simulink model "mass_spring_damper_control"  (R2022a)
settings: Solver=VariableStepAuto  StartTime=0.0  StopTime=10.0  MaxStep=1e-2  RelTol=1e-3
InitFcn:
  | start;
values from neighbouring files (symbols this model uses):
  d = 1    [start.m]
  dy0 = 0    [start.m]
  k = 2    [start.m]
  m = 1    [start.m]
  y0 = 0    [start.m]
settings Model: Creator=mathe  LastModifiedBy=mathe

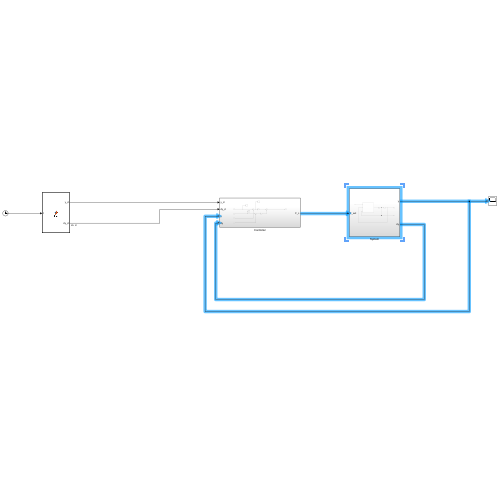
[thumbnail: Simulink's stored preview of the top-level diagram]
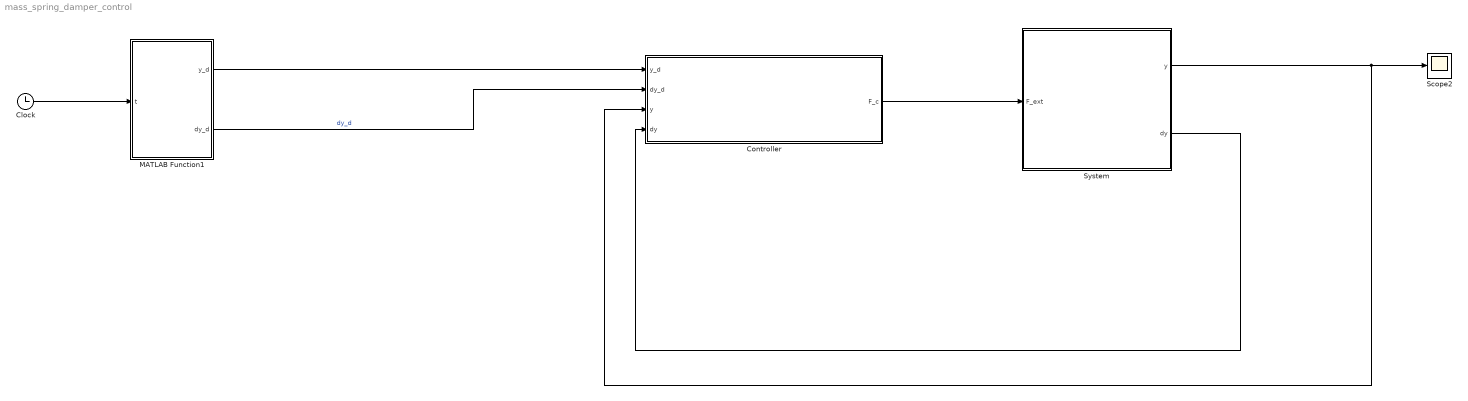
== system mass_spring_damper_control ==
  Clock : Clock
  Controller : Subsystem
  MATLAB Function1 : MATLAB Function  TreatAsAtomicUnit=on
  Scope2 : Scope
  System : Subsystem
  wires:
  Clock/1 -> MATLAB Function1/1(t)
  System/1(y) -> Controller/3(y), Scope2/1
  MATLAB Function1/1(y_d) -> Controller/1(y_d)
  System/2(dy) -> Controller/4(dy)
  MATLAB Function1/2(dy_d) -> Controller/2(dy_d)  "dy_d"
  Controller/1(F_c) -> System/1(F_ext)

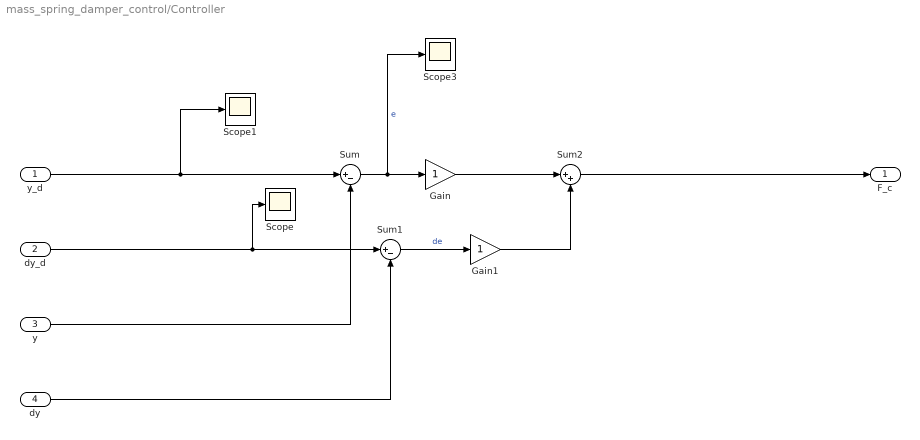
== system mass_spring_damper_control/Controller ==
  y_d : Inport
  dy_d : Inport  Port=2
  y : Inport  Port=3
  dy : Inport  Port=4
  Gain : Gain
  Gain1 : Gain
  Scope : Scope
  Scope1 : Scope
  Scope3 : Scope
  Sum : Sum  Inputs=|+-
  Sum1 : Sum  Inputs=|+-
  Sum2 : Sum  Inputs=|++
  F_c : Outport
  wires:
  Gain1/1 -> Sum2/2
  dy_d/1 -> Scope/1, Sum1/1
  Sum/1 -> Scope3/1, Gain/1  "e"
  Gain/1 -> Sum2/1
  y_d/1 -> Scope1/1, Sum/1
  Sum2/1 -> F_c/1
  Sum1/1 -> Gain1/1  "de"
  dy/1 -> Sum1/2
  y/1 -> Sum/2

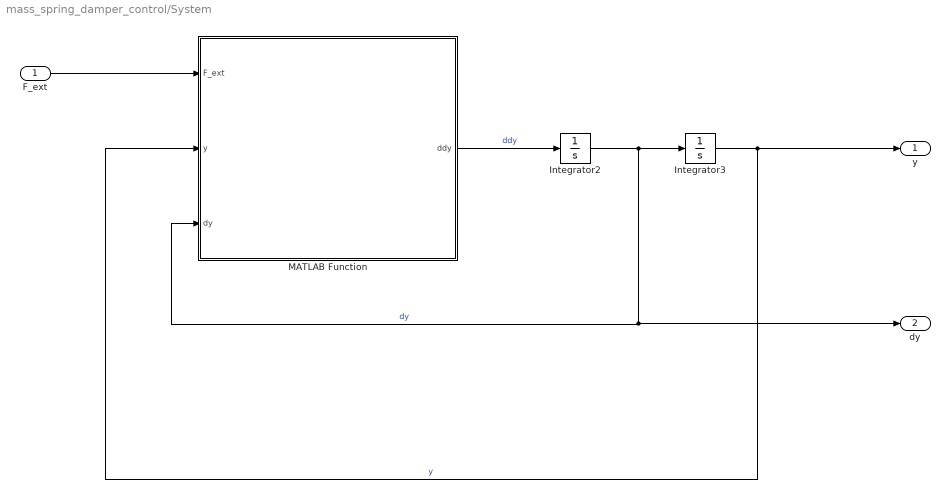
== system mass_spring_damper_control/System ==
  F_ext : Inport
  Integrator2 : Integrator  InitialCondition=dy0
  Integrator3 : Integrator  InitialCondition=y0
  MATLAB Function : MATLAB Function  TreatAsAtomicUnit=on
  y : Outport
  dy : Outport  Port=2
  wires:
  Integrator2/1 -> Integrator3/1, MATLAB Function/3(dy), dy/1  "dy"
  F_ext/1 -> MATLAB Function/1(F_ext)
  MATLAB Function/1(ddy) -> Integrator2/1  "ddy"
  Integrator3/1 -> MATLAB Function/2(y), y/1  "y"

== matlab function mass_spring_damper_control/MATLAB Function1 ==
  data: t input; y_d output; dy_d output
function [y_d, dy_d] = fcn(t)

y_d = sin(t);
dy_d = cos(t);

== matlab function mass_spring_damper_control/System/MATLAB Function ==
  data: F_ext input; ddy output; y input; dy input; m parameter; k parameter; d parameter
function ddy = fcn(F_ext, y, dy, m, k, d)

ddy = F_ext/m - d/m*dy - k/m*y;
